simulink model "PIDControl"  (R2020a)
settings: Solver=ode4  StartTime=0.0  StopTime=100  FixedStep=5e-5  RelTol=1e-3
undefined symbols (not defined in the file or in its folder): sigbuilder_block
libraries: simulink x1
settings Model: Creator=nnnmmm  LastModifiedBy=nnnmmm

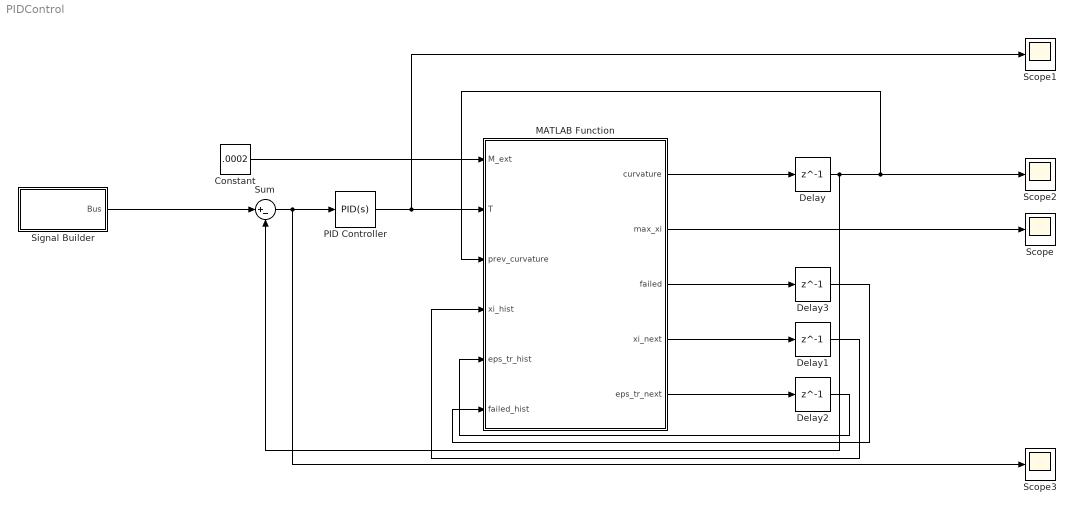
== system PIDControl ==
  Constant : Constant  Value=.0002
  Delay : Delay  DelayLength=1
  Delay1 : Delay  DelayLength=1  InitialCondition=ones(1,11)
  Delay2 : Delay  DelayLength=1  InitialCondition=zeros(1,11)
  Delay3 : Delay  DelayLength=1
  MATLAB Function : MATLAB Function  TreatAsAtomicUnit=on
  PID Controller : simulink/Continuous/PID Controller  Controller=PID  Form=Parallel  TimeDomain=Continuous-time  UseExternalTs=off  SampleTime=-1  IntegratorMethod=Forward Euler  FilterMethod=Forward Euler  ControllerParametersSource=internal  P=-.1  I=-2.2  D=0  UseFilter=on  N=100  TunerSelectOption=Transfer Function Based (PID Tuner App)  InitialConditionSource=internal  InitialConditionForIntegrator=0  InitialConditionForFilter=0  DifferentiatorICPrevScaledInput=0  ExternalReset=none  TrackingMode=off  Kt=1  LimitOutput=on  UpperSaturationLimit=350  LowerSaturationLimit=255  LinearizeAsGain=on  AntiWindupMode=clamping  Kb=1  POutMin=[]  POutMax=[]  IOutMin=[]  IOutMax=[]  DOutMin=[]  DOutMax=[]  NOutMin=[]  NOutMax=[]  SumOutMin=[]  SumOutMax=[]  SaturationOutMin=[]  SaturationOutMax=[]  PParamMin=[]  PParamMax=[]  IParamMin=[]  IParamMax=[]  DParamMin=[]  DParamMax=[]  NParamMin=[]  NParamMax=[]  KbParamMin=[]  KbParamMax=[]  KtParamMin=[]  KtParamMax=[]  KbOutMin=[]  KbOutMax=[]  KtOutMin=[]  KtOutMax=[]  IntegratorOutMin=[]  IntegratorOutMax=[]  FilterOutMin=[]  FilterOutMax=[]  SumI1OutMin=[]  SumI1OutMax=[]  SumI2OutMin=[]  SumI2OutMax=[]  SumI3OutMin=[]  SumI3OutMax=[]  SumI4OutMin=[]  SumI4OutMax=[]  SumDOutMin=[]  SumDOutMax=[]  DifferentiatorOutMin=[]  DifferentiatorOutMax=[]  FilterDiffOutCoefMin=[]  FilterDiffOutCoefMax=[]  ReciprocalOutMin=[]  ReciprocalOutMax=[]  SumDenOutMin=[]  SumDenOutMax=[]  SumNumOutMin=[]  SumNumOutMax=[]  DivideOutMin=[]  DivideOutMax=[]  UdiffTsProdOutMin=[]  UdiffTsProdOutMax=[]  NTsProdOutMin=[]  NTsProdOutMax=[]  UintegralTsProdOutMin=[]  UintegralTsProdOutMax=[]  UngainTsProdOutMin=[]  UngainTsProdOutMax=[]  IntegratorContinuousStateAttributes=''  IntegratorStateMustResolveToSignalObject=off  IntegratorRTWStateStorageClass=Auto  FilterContinuousStateAttributes=''  FilterStateMustResolveToSignalObject=off  FilterRTWStateStorageClass=Auto  ParallelPVariant=InternalParameters  IdealPVariant=Disabled  IVariant=InternalParameters  DVariant=InternalParameters  IntegratorVariant=Continuous  SatVariant=Enabled  AWVariant=ContClampingParallel  PCopyVariant=Disabled  TRVariant=Disabled  FdbkBlocksVariant=Forward  IdealPFdbkVariant=Disabled  SatFdbkVariant=Disabled  DerivativeFilterVariant=ContFilter  NVariant=InternalParameters  NCopyVariant=Disabled  FilterICVariant=InternalICsFilter  IntegratorICVariant=InternalICs  ExternalResetVariant=Disabled  TRSumVariant=Passthrough  SumFdbkVariant=Disabled  SumVariant=Sum_PID  TsampFilterVariant=InternalTs  TsampNgainVariant=Passthrough  TsampIntegralVariant=Passthrough
  Scope{,1..3} (4 alike) : Scope
  Signal Builder : Subsystem  Tag=STV Subsys  LoadFcn=sigbuilder_block('load');  StartFcn=sigbuilder_block('start');  StopFcn=sigbuilder_block('stop');  ClipboardFcn=sigbuilder_block('clipboard');  mask(Sigbuilder block){tuvar=[0:10]}
      mask help: Simulink:masks:SigbuilderBlock_MD
      mask init:
      | if ~strcmp(get_param(bdroot(gcbh),'SimulationStatus'),'stopped') tuvar = sigbuilder_block('maskInit'); end
      settings: CopyFcn=sigbuilder_block('copy');  DeleteFcn=sigbuilder_block('delete');  ModelCloseFcn=sigbuilder_block('modelClose');  PreSaveFcn=sigbuilder_block('preSave');  PauseFcn=sigbuilder_block('pause');  ContinueFcn=sigbuilder_block('continue');  NameChangeFcn=sigbuilder_block('namechange');  OpenFcn=sigbuilder_block('open',[82.2 124.2 550.8 400.2 ]);  CloseFcn=sigbuilder_block('close');
      mask Display: plot(0, 0, 100, 100,[2, 2, 32, 32, 2], [68, 8, 8, 68, 68],[32, 2], [38, 38], [32, 19, 2],[53, 60, 44], [32, 17, 17, 2],[16, 16, 31, 31]);txt = getActiveGroup(gcbh);text(2, 100, txt,'verticalAlignment', 'top');
  Sum : Sum  Inputs=|+-
  wires:
  MATLAB Function/1(curvature) -> Delay/1
  Delay/1 -> MATLAB Function/3(prev_curvature), Scope2/1, Sum/2
  MATLAB Function/4(xi_next) -> Delay1/1
  Delay1/1 -> MATLAB Function/4(xi_hist)
  MATLAB Function/5(eps_tr_next) -> Delay2/1
  Delay2/1 -> MATLAB Function/5(eps_tr_hist)
  MATLAB Function/3(failed) -> Delay3/1
  Delay3/1 -> MATLAB Function/6(failed_hist)
  MATLAB Function/2(max_xi) -> Scope/1
  Constant/1 -> MATLAB Function/1(M_ext)
  Signal Builder/1(Bus) -> Sum/1
  PID Controller/1 -> Scope1/1, MATLAB Function/2(T)
  Sum/1 -> Scope3/1, PID Controller/1

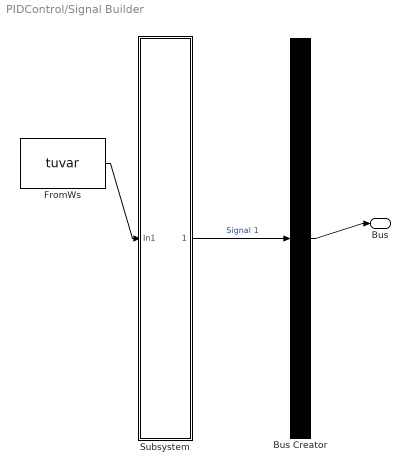
== system PIDControl/Signal Builder ==
  Bus Creator : BusCreator  Tag=Bus Creator  Inputs=1
  FromWs : FromWorkspace  Tag=STV FromWs  VariableName=tuvar
      SigBuilderData=|
      | common.afterFinalStr = 'Extrapolate'
      | common.sampleTime = 0
      | dataSet.timeRange = [0 60]
      | dataSet.name = 'Group 1'
      | sbobj.Groups.Name = 'Group 1'
      | sbobj.Groups.Signals.Name = 'Signal 1'
      | sbobj.Groups.Signals.XData = [0 14.7 14.7 40 40 60]
      | sbobj.Groups.Signals.YData = [5.5 5.5 2.5 2.5 6 6]
      | sbobj.Groups.TimeRange = [0 60]
  Subsystem : Subsystem
  Bus : Outport
  wires:
  FromWs/1 -> Subsystem/1(In1)
  Subsystem/1(Signal 1) -> Bus Creator/1  "Signal 1"
  Bus Creator/1 -> Bus/1

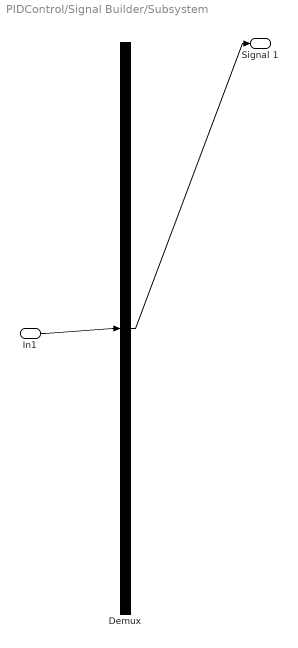
== system PIDControl/Signal Builder/Subsystem ==
  In1 : Inport
  Demux : Demux  Tag=STV Demux  Outputs=1
      settings: DisplayOption=none
  Signal 1 : Outport  Tag=STV Outport
  wires:
  Demux/1 -> Signal 1/1
  In1/1 -> Demux/1

== matlab function PIDControl/MATLAB Function ==
  data: M_ext input; T input; prev_curvature input; xi_hist input; eps_tr_hist input; curvature output; max_xi output; failed_hist input; failed output; xi_next output; eps_tr_next output
function [curvature, max_xi,  failed, xi_next, eps_tr_next] = lagoudas_wire_pure_bending(M_ext, T, prev_curvature, xi_hist, eps_tr_hist, failed_hist)
%#codegen

% =========================================================================
% ─── SIMULINK CODER INCLUSIONS: IMMEDIATE VARIABLE INITIALIZATION ───
% =========================================================================
failed = 0.0; 
curvature = 0.0;

surface_sigma = 0.0;
 % Active structural tracking for Joule heating latent math

% Strict [11 x 1] column vector properties for code generation alignment
xi_next = zeros(11, 1);
eps_tr_next = zeros(11, 1);

% =========================================================================
% 1. WIRE CROSS-SECTIONAL SLICE DISCRETIZATION (11 Symmetrical Layers)
% =========================================================================
R_wire = 0.25e-3;   % Wire radius (0.5 mm diameter)
N_layers = 11;      
y_coords = linspace(-R_wire, R_wire, N_layers); 
y_coords = y_coords(:); 
dy = y_coords(2) - y_coords(1);
dt = 0.0001;        % Explicit model timestep match

xi_current = xi_hist(:);
eps_tr_current = eps_tr_hist(:);

% =========================================================================
% 2. EXPLICIT MATERIAL LITERAL CONSTANTS (With COMSOL Internal Math)
% =========================================================================
rho = 6450;             % Density (\rho) preserved (kg/m^3)
E_A = 70e9;             % Austenite Modulus (Pa)
E_M = 30e9;             % Martensite Modulus (Pa)
H_max = 0.045;          % Max transformation strain (solid.etrmax)
sigma_failure = 1000e6; % Ultimate Tensile Strength / Failure point (1000 MPa)

Ms = 275; Mf = 256; As = 280; Af = 300;
C_A = 8e6; C_M = 8e6;   % Clausius-Clapeyron slopes (Pa/K)
n1 = 2.0; n2 = 2.0; n3 = 2.0; n4 = 2.0; 

S_A = 1 / E_A; S_M = 1 / E_M; Delta_S = S_M - S_A; 

% Pre-calculate layer areas for vectorized calculations
w_layer = 2 * sqrt(max(0, R_wire^2 - y_coords.^2));
dA = w_layer * dy;
S_curr_static = S_A + xi_current * Delta_S;

% =========================================================================
% 3. VECTORIZED EXPLICIT STATIC SOLVER LOOP FOR MECHANICAL EQUILIBRIUM
% =========================================================================
low_k = -150.0; 
high_k = 150.0; 
tol = 1e-6;
curvature = prev_curvature;

for iter = 1:60
    mid_k = (low_k + high_k) / 2;
    
    % Vectorized evaluation across all cross-section layers at once
    eps_mid = -y_coords * mid_k;
    sigma_mid = (eps_mid - eps_tr_current) ./ S_curr_static;
    M_calc_mid = sum(-sigma_mid .* y_coords .* dA);
    
    eps_low = -y_coords * low_k;
    sigma_low = (eps_low - eps_tr_current) ./ S_curr_static;
    M_calc_low = sum(-sigma_low .* y_coords .* dA);
    
    residual_mid = M_calc_mid - M_ext;
    residual_low = M_calc_low - M_ext;
    
    if abs(residual_mid) < tol
        curvature = mid_k;
        break;
    end
    
    if (residual_low * residual_mid) < 0
        high_k = mid_k;
    else
        low_k = mid_k;
    end
end

% Ensure curvature falls back to the final bisection point if tol isn't met
if abs(residual_mid) >= tol
    curvature = (low_k + high_k) / 2;
end

% =========================================================================
% 4. LAYER PROGRESSION UPDATE WITH EXPLICIT RELAXATION FILTERING
% =========================================================================
sigma_max_track = 0.0;
xi_unfiltered = zeros(N_layers, 1);

for j = 1:N_layers
    epsilon = -y_coords(j) * curvature;
    S_curr = S_A + xi_current(j) * Delta_S;
    sigma_layer = (epsilon - eps_tr_current(j)) / S_curr;
    
    if abs(sigma_layer) > sigma_max_track
        sigma_max_track = abs(sigma_layer);
    end
    
    sgn_sig = sign(sigma_layer);
    if sgn_sig == 0; sgn_sig = 1; end
    
    Ms_s = Ms + abs(sigma_layer) / C_M;
    Mf_s = Mf + abs(sigma_layer) / C_M;
    As_s = As + abs(sigma_layer) / C_A;
    Af_s = Af + abs(sigma_layer) / C_A;
    
    xi_target = xi_current(j); 
    
    if abs(curvature) > 0.005
        if (T < Ms_s) && (T > Mf_s)
            linear_ratio = (T - Mf_s) / (Ms_s - Mf_s);
            trial_target = 1.0 - (linear_ratio^n1 / (linear_ratio^n1 + (1.0 - linear_ratio)^n2));
            if trial_target > xi_current(j); xi_target = trial_target; end
        elseif T <= Mf_s
            xi_target = 1.0;
        end
        
        if (T > As_s) && (T < Af_s)
            linear_ratio = (T - As_s) / (Af_s - As_s);
            trial_target = 1.0 - (linear_ratio^n3 / (linear_ratio^n3 + (1.0 - linear_ratio)^n4));
            if trial_target < xi_current(j); xi_target = trial_target; end
        elseif T >= Af_s
            xi_target = 0.0;
        end
    else
        if T > Af; xi_target = 0.0; elseif T < Mf; xi_target = 1.0; end
    end
    
    xi_unfiltered(j) = xi_target;
    
    % Balanced relaxation factor (Increased to 5% for realistic heat transient calculations)
    xi_current(j) = xi_hist(j) + 0.05 * (xi_target - xi_hist(j));
    
    sigma_detwin = 70e6;
    if abs(sigma_layer) > 1e-3
        detwin_factor = min(1.0, abs(sigma_layer) / sigma_detwin);
        eps_tr_target = sgn_sig * H_max * xi_current(j) * detwin_factor;
    else
        eps_tr_target = 0.0;
    end
    
    eps_tr_current(j) = eps_tr_hist(j) + 0.05 * (eps_tr_target - eps_tr_hist(j));
end

% Check failure limit against material properties
if sigma_max_track > sigma_failure
    failed = 1.0;
end

% =========================================================================
% 5. ASSIGN FINAL OUTPUT PARAMETERS
% =========================================================================
max_xi = max(xi_current);
surface_sigma = sigma_max_track;

% Extract a true, non-damped structural derivative for the latent heat model
mean_xi_target = mean(xi_unfiltered);
mean_xi_hist = mean(xi_hist);
dxi_dt = (mean_xi_target - mean_xi_hist) / dt;

xi_next = xi_current(:);
eps_tr_next = eps_tr_current(:);

end
